simulink model "simple"  (Simulink 7.9)
settings: Solver=ode45  StartTime=0.0  StopTime=10  RelTol=1e-3
libraries: simulink x1, truetime x1
settings Model: Creator=anton  LastModifiedBy=mogaf  ExtModeAutoUpdateStatusClock=off
settings OptimizationCC: BooleanDataType=off
settings DebuggingCC: SaveWithParameterizedLinksMsg=none  SignalResolutionControl=TryResolveAllWithWarning  SolverPrmCheckMsg=none  MultiTaskDSMMsg=warning  MultiTaskCondExecSysMsg=none  StrictBusMsg=None
settings HardwareCC: TargetUnknown=on
settings RTWCC: IncludeERTFirstTime=on
settings GRTTargetCC: CombineOutputUpdateFcns=off  GRTInterface=on

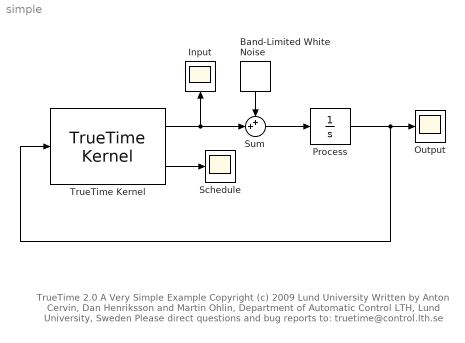
== system simple ==
  note: TrueTime 2.0  A Very Simple Example
      | Copyright (c) 2009 Lund University
      | Written by Anton Cervin, Dan Henriksson and Martin Ohlin,
      | Department of Automatic Control LTH, Lund University, Sweden
      | Please direct questions and bug reports to: truetime@control.lth.se
  Band-Limited White Noise : simulink/Sources/Band-Limited White Noise  Cov=[0.1]  Ts=0.1  seed=[23341]
  Input : Scope
      settings: TimeRange=10  YMin=-1  YMax=1  SaveName=ScopeData2
  Output : Scope
      settings: TimeRange=10  YMin=-1  YMax=1
  Process : Integrator
  Schedule : Scope
      settings: YMin=0  YMax=2
  Sum : Sum  Inputs=++|  SaturateOnIntegerOverflow=on  InputSameDT=on  OutDataTypeStr=Inherit: Same as first input
  TrueTime Kernel : truetime/TrueTime Kernel  sfun=simple_init  args=[]  ninputsoutputs=[1 1]  ntriggers=0  trigtype=falling  nwnodenbr=[]  clockoffsetdrift=[0 0]  schedoutput=on  battery=off  poweroutput=off
  wires:
  TrueTime Kernel/2 -> Schedule/1
  TrueTime Kernel/1 -> Input/1, Sum/2
  Process/1 -> Output/1, TrueTime Kernel/1
  Sum/1 -> Process/1
  Band-Limited White Noise/1 -> Sum/1
